simulink model "cruise_control_aberta"  (R2020b)
settings: Solver=VariableStepAuto  StartTime=0.0  StopTime=100.0  FixedStep=1e-3  RelTol=1e-3
undefined symbols (not defined in the file or in its folder): b, d, m
settings Model: Creator=mmaximo  LastModifiedBy=kenji

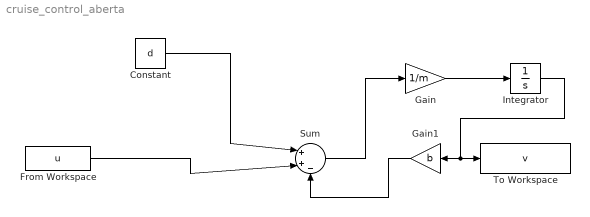
== system cruise_control_aberta ==
  Constant : Constant  Value=d
  From Workspace : FromWorkspace  VariableName=u
  Gain : Gain  Gain=1/m
  Gain1 : Gain  Gain=b
  Integrator : Integrator
  Sum : Sum  Inputs=|++-
  To Workspace : ToWorkspace  VariableName=v  SaveFormat=Structure With Time  SampleTime=-1
  wires:
  From Workspace/1 -> Sum/2
  Constant/1 -> Sum/1
  Sum/1 -> Gain/1
  Gain/1 -> Integrator/1
  Integrator/1 -> To Workspace/1, Gain1/1
  Gain1/1 -> Sum/3
